simulink model "Pract5_fin"  (Simulink 8.4)
settings: Solver=ode45  StartTime=0.0  StopTime=0.01  RelTol=1e-3
libraries: simulink x4, dspsigops x3, commnoisgen2 x1, commrandsrc2 x1
settings Model: Creator=Labcom  LastModifiedBy=mazo2

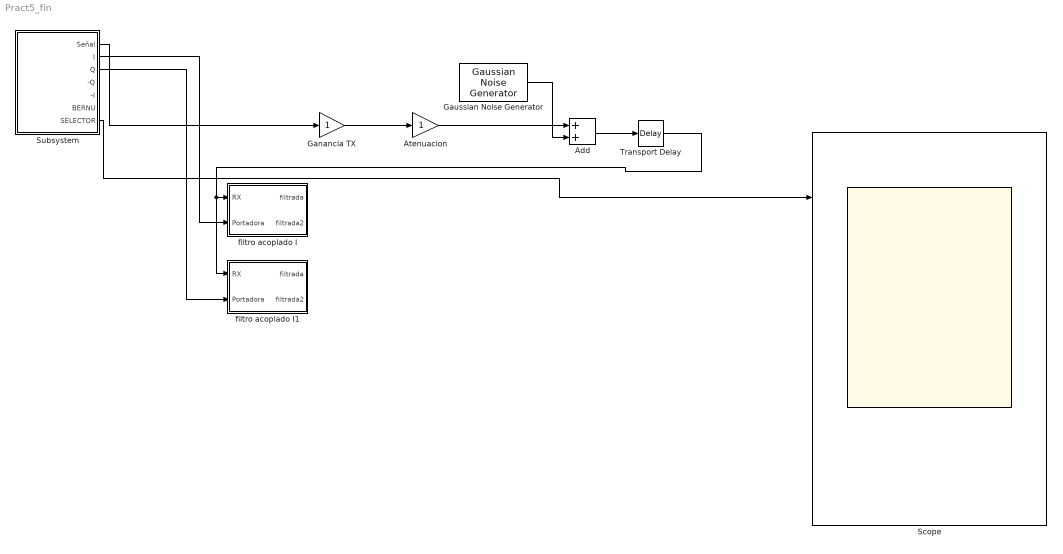
== system Pract5_fin ==
  Add : Sum
  Atenuacion : Gain
  Ganancia TX : Gain
  Gaussian Noise Generator : commnoisgen2/Gaussian Noise Generator  m=0  d=0  s=41  Ts=0.00000001  frameBased=off  sampPerFrame=1  orient=off  outDataType=double
  Scope : Scope  NumInputPorts=3
      settings: TickLabels=on  TimeRange=0.01  YMin=0~-0.1~-110  YMax=3.5~1.5~110  MaxDataPoints=100000
  Subsystem : Subsystem
  Transport Delay : TransportDelay  DelayTime=0
  filtro acoplado I : Subsystem
  filtro acoplado I1 : Subsystem
  wires:
  Add/1 -> Transport Delay/1
  Atenuacion/1 -> Add/1
  Ganancia TX/1 -> Atenuacion/1
  Gaussian Noise Generator/1 -> Add/2
  Transport Delay/1 -> filtro acoplado I1/1(RX), filtro acoplado I/1(RX)
  Subsystem/1(Señal) -> Ganancia TX/1
  Subsystem/2(I) -> filtro acoplado I/2(Portadora)
  Subsystem/3(Q) -> filtro acoplado I1/2(Portadora)
  Subsystem/7(SELECTOR) -> Scope/1

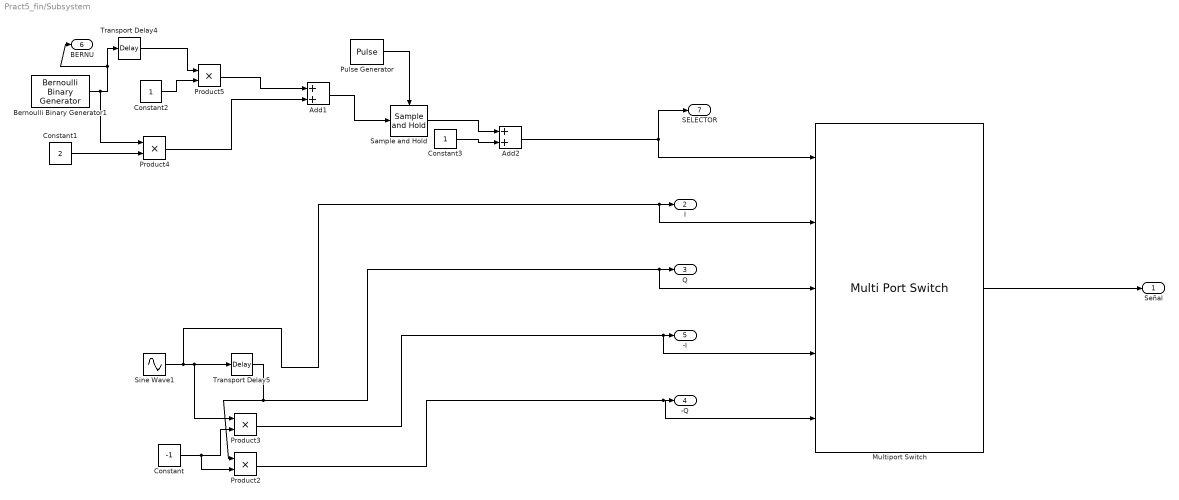
== system Pract5_fin/Subsystem ==
  Add1 : Sum
  Add2 : Sum
  Bernoulli Binary Generator1 : commrandsrc2/Bernoulli Binary Generator  P=0.5  seed=35  Ts=0.0005  frameBased=off  sampPerFrame=1  orient=off  outDataType=double
  Constant : Constant  Value=-1
  Constant1 : Constant  Value=2
  Constant2 : Constant
  Constant3 : Constant
  Multiport Switch : MultiPortSwitch  Inputs=4
  Product{2..5} (4 alike) : Product  RndMeth=Zero
  Pulse Generator : DiscretePulseGenerator  PulseType=Time based  Period=0.001  PulseWidth=99
  Sample and Hold : dspsigops/Sample and Hold  trig=Falling edge  initCond=0  latchinput=off
  Sine Wave1 : Sin  Frequency=2*pi*1000000  SampleTime=0.00000001
  Transport Delay4 : TransportDelay  DelayTime=0.0005
  Transport Delay5 : TransportDelay  DelayTime=0.000001/4
  Señal : Outport
  I : Outport  Port=2
  Q : Outport  Port=3
  -Q : Outport  Port=4
  -I : Outport  Port=5
  BERNU : Outport  Port=6
  SELECTOR : Outport  Port=7
  wires:
  Sine Wave1/1 -> Transport Delay5/1, Product3/1, I/1, Multiport Switch/2
  Constant/1 -> Product3/2, Product2/2
  Bernoulli Binary Generator1/1 -> Product4/1, Transport Delay4/1, BERNU/1
  Product3/1 -> Multiport Switch/4, -I/1
  Product2/1 -> Multiport Switch/5, -Q/1
  Transport Delay4/1 -> Product5/1
  Constant1/1 -> Product4/2
  Constant2/1 -> Product5/2
  Product5/1 -> Add1/1
  Product4/1 -> Add1/2
  Constant3/1 -> Add2/2
  Add2/1 -> SELECTOR/1, Multiport Switch/1
  Multiport Switch/1 -> Señal/1
  Add1/1 -> Sample and Hold/1
  Sample and Hold/1 -> Add2/1
  Pulse Generator/1 -> Sample and Hold/Trigger
  Transport Delay5/1 -> Product2/1, Q/1, Multiport Switch/3

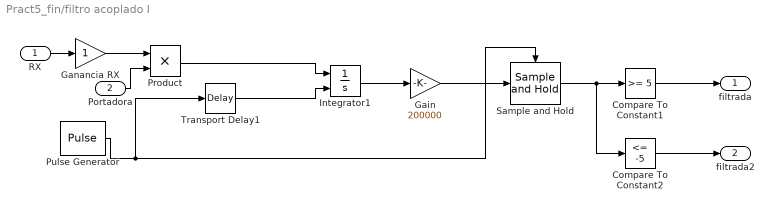
== system Pract5_fin/filtro acoplado I ==
  RX : Inport
  Portadora : Inport  Port=2
  Compare To Constant1 : simulink/Logic and Bit Operations/Compare To Constant  relop=>=  const=5  OutDataTypeStr=uint8  ZeroCross=off
  Compare To Constant2 : simulink/Logic and Bit Operations/Compare To Constant  relop=<=  const=-5  OutDataTypeStr=uint8  ZeroCross=off
  Gain : Gain  Gain=200000
  Ganancia RX : Gain
  Integrator1 : Integrator  ExternalReset=falling  UpperSaturationLimit=1  LowerSaturationLimit=0
  Product : Product  RndMeth=Zero
  Pulse Generator : DiscretePulseGenerator  PulseType=Time based  Period=0.001  PulseWidth=99
  Sample and Hold : dspsigops/Sample and Hold  trig=Falling edge  initCond=0  latchinput=off
  Transport Delay1 : TransportDelay  DelayTime=0.0000003
  filtrada : Outport
  filtrada2 : Outport  Port=2
  wires:
  Integrator1/1 -> Gain/1
  Gain/1 -> Sample and Hold/1
  Pulse Generator/1 -> Sample and Hold/Trigger, Transport Delay1/1
  Ganancia RX/1 -> Product/1
  Product/1 -> Integrator1/1
  Transport Delay1/1 -> Integrator1/2
  RX/1 -> Ganancia RX/1
  Portadora/1 -> Product/2
  Compare To Constant1/1 -> filtrada/1
  Sample and Hold/1 -> Compare To Constant2/1, Compare To Constant1/1
  Compare To Constant2/1 -> filtrada2/1

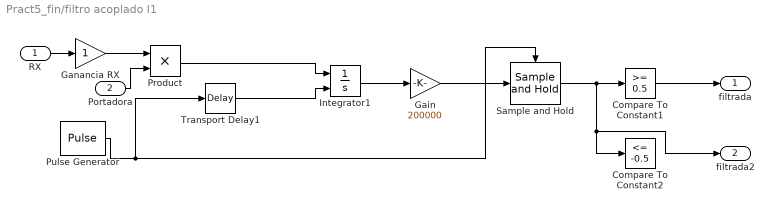
== system Pract5_fin/filtro acoplado I1 ==
  RX : Inport
  Portadora : Inport  Port=2
  Compare To Constant1 : simulink/Logic and Bit Operations/Compare To Constant  relop=>=  const=0.5  OutDataTypeStr=uint8  ZeroCross=off
  Compare To Constant2 : simulink/Logic and Bit Operations/Compare To Constant  relop=<=  const=-0.5  OutDataTypeStr=uint8  ZeroCross=off
  Gain : Gain  Gain=200000
  Ganancia RX : Gain
  Integrator1 : Integrator  ExternalReset=falling  UpperSaturationLimit=1  LowerSaturationLimit=0
  Product : Product  RndMeth=Zero
  Pulse Generator : DiscretePulseGenerator  PulseType=Time based  Period=0.001  PulseWidth=99
  Sample and Hold : dspsigops/Sample and Hold  trig=Falling edge  initCond=0  latchinput=off
  Transport Delay1 : TransportDelay  DelayTime=0.0000003
  filtrada : Outport
  filtrada2 : Outport  Port=2
  wires:
  Integrator1/1 -> Gain/1
  Gain/1 -> Sample and Hold/1
  Pulse Generator/1 -> Sample and Hold/Trigger, Transport Delay1/1
  Ganancia RX/1 -> Product/1
  Product/1 -> Integrator1/1
  Transport Delay1/1 -> Integrator1/2
  RX/1 -> Ganancia RX/1
  Portadora/1 -> Product/2
  Compare To Constant1/1 -> filtrada/1
  Sample and Hold/1 -> Compare To Constant2/1, filtrada2/1, Compare To Constant1/1
